simulink model "EV_Modeling"  (R2024b)
settings: Solver=FixedStepAuto  StartTime=0.0  StopTime=3500  FixedStep=0.1  RelTol=1e-3
values from neighbouring files (symbols this model uses):
  battery_SOC_resistance = battery_SOC(:,3)    [EV_Truck.m]
  battery_SOC_SOC = battery_SOC(:,1)    [EV_Truck.m]    (also in simulink.m)
  battery_SOC_voltage = battery_SOC(:,2)    [EV_Truck.m]    (also in simulink.m)
  electric_consumption_ressistancce = electric_consumption(:,2)    [EV_Truck.m]    (also in simulink.m)
  electric_consumption_voltage = electric_consumption(:,1)    [EV_Truck.m]    (also in simulink.m)
  motor_efficiency_efficiency = table2array(motor_efficiency(2:height(motor_efficiency),2:width(motor_efficiency)))    [EV_Truck.m]    (also in simulink.m)
  motor_efficiency_RPM = table2array(motor_efficiency(2:height(motor_efficiency),1))    [EV_Truck.m]    (also in simulink.m)
  motor_efficiency_torque = transpose(motor_efficiency_torque)    [EV_Truck.m]    (also in simulink.m)
  motor_RPM_torque = table2array(motor_torque(1:14,1))    [EV_Truck.m]    (also in simulink.m)
  motor_torque_RPM = table2array(motor_torque(1:14,2))    [EV_Truck.m]    (also in simulink.m)
undefined symbols (not defined in the file or in its folder): battery_builder_rtmsupport, battery_sli_rtmsupport, DiscIntNeverNeededParam, gcbh, recurrentNet
libraries: dlutilitylib x10, dlsequencelib x10, packLibrary_lib x10, simulink x7, dlconvfclib x6, dlactivationlib x5, sharedTrackingLibrary x3, mpcadaslib x2, nesl_utility x2, fl_lib x2, slpidlib x2, simulink_extras x1
(part 1 of 9)
settings Model: SILPILSystemUnderTest=refmodels  Creator=Administrator  LastModifiedBy=avees
settings SolverCC: AlgebraicLoopSolver=TrustRegion
settings DataIOCC: ExternalInput=EV_ModelingScenario.getElement('Input')
settings OptimizationCC: DefaultParameterBehavior=Inlined  UseDivisionForNetSlopeComputation=on  GainParamInheritBuiltInType=on  UseFloatMulNetSlope=on  UseSpecifiedMinMax=on  InlineInvariantSignals=on  PassReuseOutputArgsAs=Individual arguments  ZeroExternalMemoryAtStartup=off  ZeroInternalMemoryAtStartup=off  NoFixptDivByZeroProtection=on  EfficientFloat2IntCast=on  LifeSpan=1  OptimizeBlockOrder=speed  DifferentSizesBufferReuse=on  EfficientTunableParamExpr=on
settings DebuggingCC: ParameterTunabilityLossMsg=error  UnconnectedInputMsg=warning  UnconnectedOutputMsg=warning  UnconnectedLineMsg=warning
settings HardwareCC: ProdBitPerLong=64  ProdLargestAtomicInteger=LongLong  ProdLargestAtomicFloat=Double  ProdLongLongMode=on  ProdHWDeviceType=ARM Compatible->ARM Cortex-A (64-bit)
settings ModelReferenceCC: EnableRefExpFcnMdlSchedulingChecks=on
settings SFSimCC: MATLABDynamicMemAlloc=off  SimTargetLang=C++
settings RTWCC: Description=Embedded Coder  SystemTargetFile=ert.tlc  GenCodeOnly=on  TemplateMakefile=ert_default_tmf  BuildConfiguration=Faster Runs  DataTypeReplacement=CDataTypesFixedWidth  TargetLang=C++  GPUComputeCapability=3.5  DLArmComputeVersion=19.05
settings CodeAppCC: ForceParamTrailComments=on  IgnoreCustomStorageClasses=off  OperatorAnnotations=on  SimulinkDataObjDesc=on  SFDataObjDesc=on  CustomSymbolStrGlobalVar=rt$N$M  CustomSymbolStrType=$N$M  CustomSymbolStrFcn=$N$M$F  CustomSymbolStrMacro=$N$M  InsertBlockDesc=on
settings ERTTargetCC: TargetLangStandard=C++11 (ISO)  GenerateSampleERTMain=on  IncludeMdlTerminateFcn=off  CombineSignalStateStructs=on  CodeInterfacePackaging=C++ class  SupportComplex=off  SupportContinuousTime=on  SupportNonInlinedSFcns=on  RootIOFormat=Structure reference  ERTCustomFileTemplate=example_file_process.tlc  ERTFilePackagingFormat=CompactWithDataFile  MaxIdInt64=INT64_MAX  MinIdInt64=INT64_MIN  MaxIdUint64=UINT64_MAX  MaxIdInt32=INT32_MAX  MinIdInt32=INT32_MIN  MaxIdUint32=UINT32_MAX  MaxIdInt16=INT16_MAX  MinIdInt16=INT16_MIN  MaxIdUint16=UINT16_MAX  MaxIdInt8=INT8_MAX  MinIdInt8=INT8_MIN  MaxIdUint8=UINT8_MAX

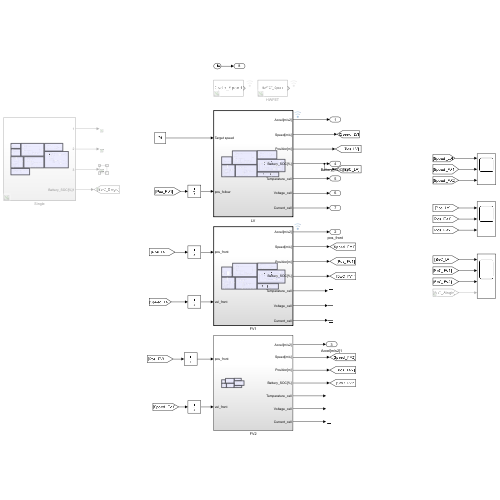
[thumbnail: Simulink's stored preview of the top-level diagram]
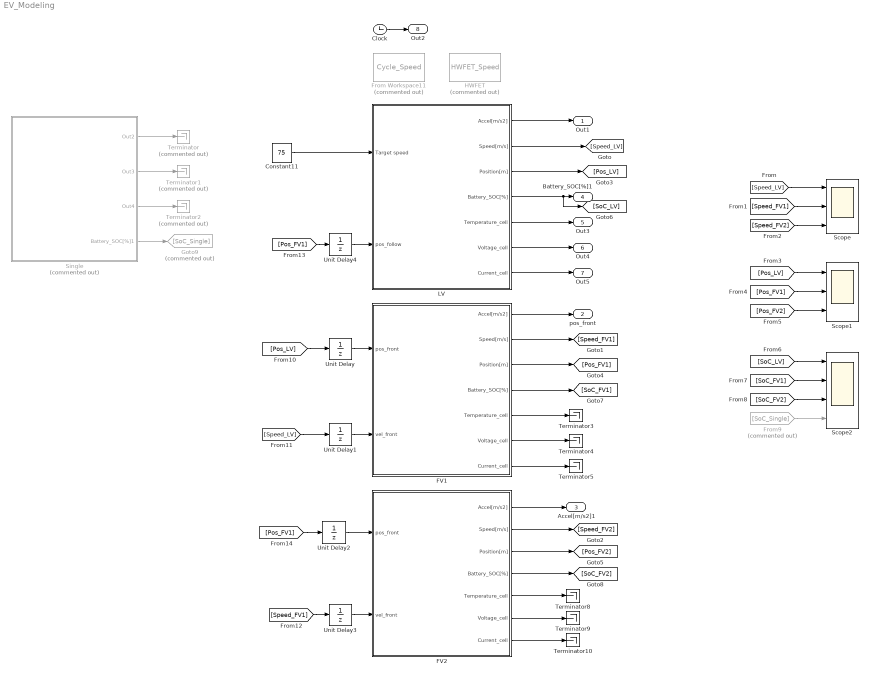
== system EV_Modeling ==
  Clock : Clock
  Constant11 : Constant  Value=75
  FV1 : Subsystem  TreatAsAtomicUnit=on
  FV2 : Subsystem
  From Workspace11 : FromWorkspace  Commented=on  VariableName=Cycle_Speed
  From9 : From  Commented=on  GotoTag=SoC_Single
  Goto9 : Goto  Commented=on  GotoTag=SoC_Single
  HWFET : FromWorkspace  Commented=on  VariableName=HWFET_Speed
  LV : Subsystem  TreatAsAtomicUnit=on
  Scope : Scope  NumInputPorts=3
  Scope1 : Scope  NumInputPorts=3
  Scope2 : Scope  NumInputPorts=4
  Single : Subsystem  Commented=on
  Terminator : Terminator  Commented=on
  Terminator1 : Terminator  Commented=on
  Terminator{3..5,8..10} (6 alike) : Terminator
  Terminator2 : Terminator  Commented=on
  Unit Delay{,1..4} (5 alike) : UnitDelay  SampleTime=-1  HasFrameUpgradeWarning=on
  Out1 : Outport
  pos_front : Outport  Port=2
  Accel[m/s2]1 : Outport  Port=3
  Battery_SOC[%]1 : Outport  Port=4
  Out3 : Outport  Port=5
  Out4 : Outport  Port=6
  Out5 : Outport  Port=7
  Out2 : Outport  Port=8
  wires:
  Constant11/1 -> LV/1(Target speed)
  LV/3(Position[m]) -> [Pos_LV]
  LV/2(Speed[m/s]) -> [Speed_LV]
  LV/1(Accel[m/s2]) -> Out1/1
  FV2/1(Accel[m/s2]) -> Accel[m/s2]1/1
  FV1/1(Accel[m/s2]) -> pos_front/1
  FV1/3(Position[m]) -> [Pos_FV1]
  FV1/2(Speed[m/s]) -> [Speed_FV1]
  [Speed_LV] -> Scope/1
  [Speed_FV1] -> Scope/2
  FV2/2(Speed[m/s]) -> [Speed_FV2]
  [Speed_FV2] -> Scope/3
  FV2/3(Position[m]) -> [Pos_FV2]
  [Pos_LV] -> Scope1/1
  [Pos_FV1] -> Scope1/2
  [Pos_FV2] -> Scope1/3
  LV/4(Battery_SOC[%]) -> [SoC_LV], Battery_SOC[%]1/1
  FV1/4(Battery_SOC[%]) -> [SoC_FV1]
  FV2/4(Battery_SOC[%]) -> [SoC_FV2]
  [SoC_LV] -> Scope2/1
  [SoC_FV1] -> Scope2/2
  [SoC_FV2] -> Scope2/3
  Single/4(Battery_SOC[%]1) -> Goto9/1
  From9/1 -> Scope2/4
  [Pos_LV] -> Unit Delay/1
  [Speed_LV] -> Unit Delay1/1
  [Speed_FV1] -> Unit Delay3/1
  [Pos_FV1] -> Unit Delay2/1
  [Pos_FV1] -> Unit Delay4/1
  LV/5(Temperature_cell) -> Out3/1
  LV/6(Voltage_cell) -> Out4/1
  LV/7(Current_cell) -> Out5/1
  Single/3(Out4) -> Terminator2/1
  Single/2(Out3) -> Terminator1/1
  Single/1(Out2) -> Terminator/1
  FV1/7(Current_cell) -> Terminator5/1
  FV1/6(Voltage_cell) -> Terminator4/1
  FV1/5(Temperature_cell) -> Terminator3/1
  FV2/6(Voltage_cell) -> Terminator9/1
  FV2/5(Temperature_cell) -> Terminator8/1
  FV2/7(Current_cell) -> Terminator10/1
  Unit Delay/1 -> FV1/1(pos_front)
  Unit Delay1/1 -> FV1/2(vel_front)
  Unit Delay2/1 -> FV2/1(pos_front)
  Unit Delay3/1 -> FV2/2(vel_front)
  Unit Delay4/1 -> LV/2(pos_follow)
  Clock/1 -> Out2/1
